simulink model "test_controller_design"  (Simulink 4.00)
settings: Solver=FixedStepDiscrete  StartTime=0.0  StopTime=100  FixedStep=0.05  RelTol=1e-3
undefined symbols (not defined in the file or in its folder): parameters
libraries: simulink3 x2, controller_design_lib x1, IdInput_block_lib x1, save_blocks_lib x1
settings Model: LastModifiedBy=bsaunder

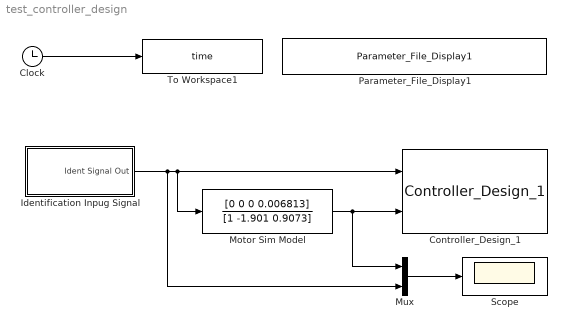
== system test_controller_design ==
  Clock : Clock
      settings: DisplayTime=off  Decimation=10
  Controller_Design_1 : controller_design_lib/Controller_Design_1  cntr_orders=parameters.motor_control_design.orders  ctrObs_dyn=parameters.motor_control_design.control_observer_dynamics  refMdl_dyn=parameters.motor_control_design.reference_model_dynamics  Ts=parameters.motor_control_design.sample_time
  Identification Inpug Signal : Subsystem
      settings: RTWFcnNameOpts=Auto  RTWFileNameOpts=Auto
  Motor Sim Model : DiscreteFilter  Numerator=[0 0 0 0.006813]  Denominator=[1 -1.901 0.9073]  SampleTime=0.05  Realization=auto
      settings: RTWStateStorageClass=Auto
  Mux : Mux  Inputs=2
  Parameter_File_Display1 : save_blocks_lib/Parameter_File_Display1
  Scope : Scope
      settings: TimeRange=auto  YMin=0  YMax=120  SaveToWorkspace=off  SaveName=ScopeData  LimitDataPoints=on  MaxDataPoints=5000
  To Workspace1 : ToWorkspace  VariableName=time  SampleTime=parameters.sample_time  SaveFormat=Array
  wires:
  Identification Inpug Signal/1(Ident Signal Out) -> Motor Sim Model/1, Controller_Design_1/1, Mux/2
  Mux/1 -> Scope/1
  Motor Sim Model/1 -> Mux/1, Controller_Design_1/2
  Clock/1 -> To Workspace1/1

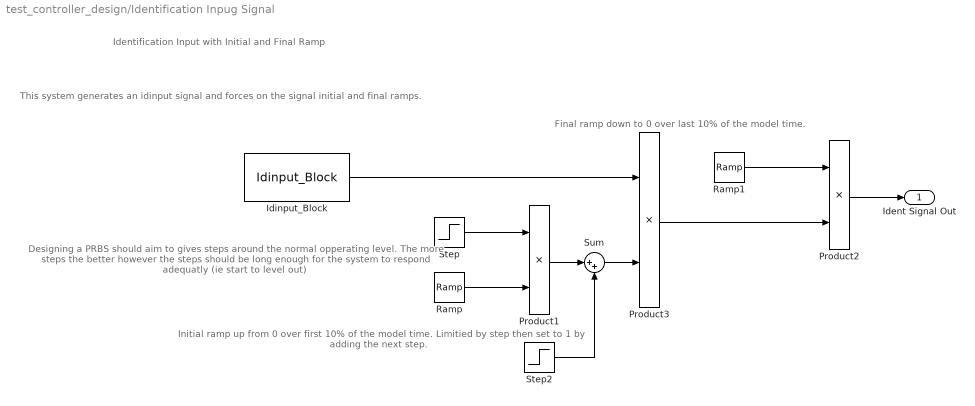
== system test_controller_design/Identification Inpug Signal ==
  note: Designing a PRBS should aim
      | to gives steps around the normal
      | opperating level.  The more
      | steps the better however the
      | steps should be long enough for
      | the system to respond adequatly
      | (ie start to level out)
  note: Identification Input with Initial and Final Ramp
  note: This system generates an
      | idinput signal and forces on
      | the signal initial and final
      | ramps.
  note: Final ramp down to 0 over last
      | 10% of the model time.
  note: Initial ramp up from 0 over
      | first 10% of the model time.
      | Limitied by step then set to
      | 1 by adding the next step.
  Idinput_Block : IdInput_block_lib/Idinput_Block  ssT=[0.1*parameters.motor_identification.total_time 0.9*parameters.motor_identification.total_time]  signal_type=PRBS  band=[0 1/parameters.motor_PRBS.min_same_time]  levels=parameters.motor_PRBS.output_limits  Ts=parameters.sample_time
  Product1 : Product  Inputs=2  Multiplication=Element-wise(.*)  SaturateOnIntegerOverflow=on
  Product2 : Product  Inputs=2  Multiplication=Element-wise(.*)  SaturateOnIntegerOverflow=on
  Product3 : Product  Inputs=2  Multiplication=Element-wise(.*)  SaturateOnIntegerOverflow=on
  Ramp : simulink3/Sources/Ramp  slope=1/(0.1 * parameters.motor_identification.total_time)  start=0  X0=0
  Ramp1 : simulink3/Sources/Ramp  slope=-(1 / (0.1 * parameters.motor_identification.total_time))  start=0.9 * parameters.motor_identification.total_time  X0=1
  Step : Step  Time=0.1 * parameters.motor_identification.total_time  Before=1  After=0  SampleTime=parameters.sample_time
  Step2 : Step  Time=0.1 * parameters.motor_identification.total_time  Before=0  After=1  SampleTime=parameters.sample_time
  Sum : Sum  Inputs=|++  SaturateOnIntegerOverflow=on
  Ident Signal Out : Outport  Port=1
  wires:
  Idinput_Block/1 -> Product3/1
  Ramp1/1 -> Product2/1
  Product2/1 -> Ident Signal Out/1
  Step/1 -> Product1/1
  Ramp/1 -> Product1/2
  Product1/1 -> Sum/1
  Sum/1 -> Product3/2
  Step2/1 -> Sum/2
  Product3/1 -> Product2/2
